simulink library "turbine_generator_v0"  (R2025b)
settings: Solver=VariableStepAuto  StartTime=0.0  StopTime=10.0  RelTol=1e-3
undefined symbols (not defined in the file): gen_eta, kT, kV, R_load, Rm, turbine_D
libraries: simulink x2
settings Model: Creator=Carson  LastModifiedBy=Carson
settings RTWCC: GPUComputeCapability=3.5

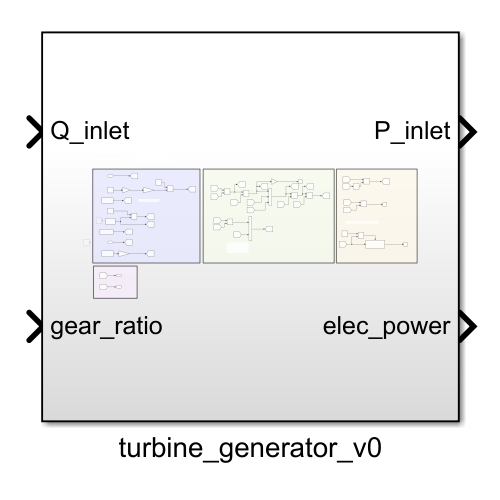
[thumbnail: Simulink's stored preview of the top-level diagram]
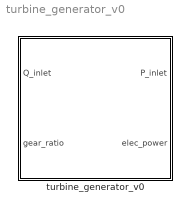
== system turbine_generator_v0 ==
  turbine_generator_v0 : Subsystem

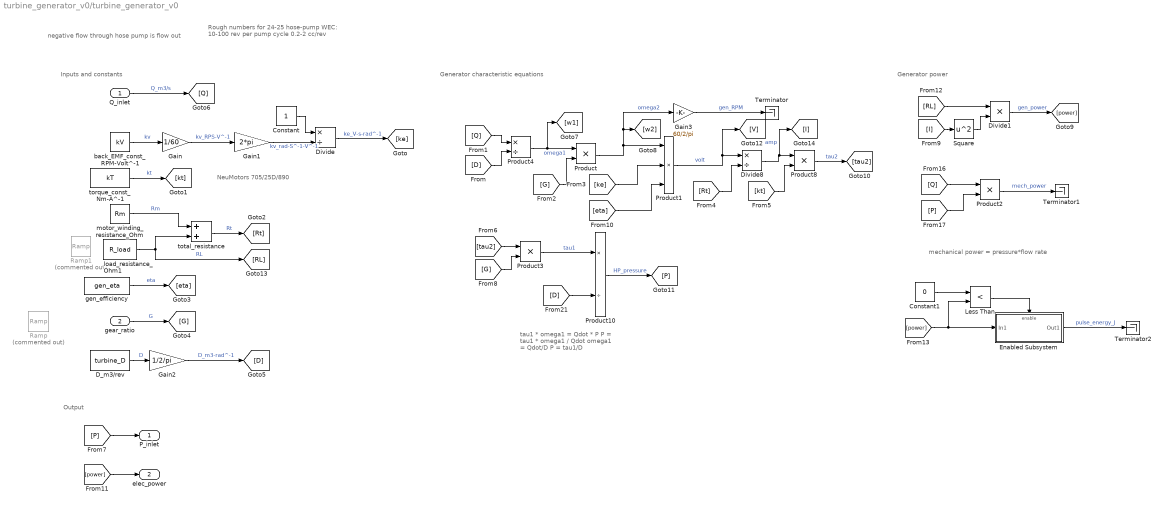
== system turbine_generator_v0/turbine_generator_v0 ==
  note: tau1 * omega1 = Qdot * P
      | P = tau1 * omega1 / Qdot
      | 	omega1 = Qdot/D
      | P = tau1/D
  note: NeuMotors 705/25D/890
  note: mechanical power = pressure*flow rate
  note: Rough numbers for 24-25 hose-pump WEC:
      | 	10-100 rev per pump cycle
      | 	0.2-2 cc/rev
  note: Generator power
  note: Output
  note: Generator characteristic equations
  note: Inputs and constants
  note: negative flow through hose pump is flow out
  Q_inlet : Inport
  gear_ratio : Inport  Port=2
  Constant : Constant
  Constant1 : Constant  Value=0
  D_m3/rev : Constant  Value=turbine_D
  Divide : Product  Inputs=*/
  Divide1 : Product  Inputs=**
  Divide8 : Product  Inputs=*/
  Enabled Subsystem : Subsystem  TreatAsAtomicUnit=on
  Gain : Gain  Gain=1/60
  Gain1 : Gain  Gain=2*pi
  Gain2 : Gain  Gain=1/2/pi
  Gain3 : Gain  Gain=60/2/pi
  Less Than : RelationalOperator  Operator=<  OutDataTypeStr=boolean  RndMeth=Simplest  InputSameDT=off
  Product{,2..3,8} (4 alike) : Product
  Product1 : Product  Inputs=3
  Product10 : Product  Inputs=*/
  Product4 : Product  Inputs=*/
  Ramp : simulink/Sources/Ramp  Commented=on  slope=0.1  start=60  InitialOutput=1
  Ramp1 : simulink/Sources/Ramp  Commented=on  slope=3/600  start=30  InitialOutput=0
  Square : Math  Operator=square
  Terminator : Terminator
  Terminator1 : Terminator
  Terminator2 : Terminator
  back_EMF_const_RPM-Volt^-1 : Constant  Value=kV
  gen_efficiency : Constant  Value=gen_eta
  load_resistance_Ohm1 : Constant  Value=R_load
  motor_winding_resistance_Ohm : Constant  Value=Rm
  torque_const_Nm-A^-1 : Constant  Value=kT
  total_resistance : Sum
  P_inlet : Outport
  elec_power : Outport  Port=2
  wires:
  torque_const_Nm-A^-1/1 -> [kt]  "kt"
  gen_efficiency/1 -> [eta]  "eta"
  motor_winding_resistance_Ohm/1 -> total_resistance/1  "Rm"
  load_resistance_Ohm1/1 -> total_resistance/2, [RL]  "RL"
  total_resistance/1 -> [Rt]  "Rt"
  Gain/1 -> Gain1/1  "kv_RPS-V^-1"
  Gain1/1 -> Divide/2  "kv_rad-S^-1-V^-1"
  Constant/1 -> Divide/1
  Divide/1 -> [ke]  "ke_V-s-rad^-1"
  D_m3/rev/1 -> Gain2/1  "D"
  Gain2/1 -> [D]  "D_m3-rad^-1"
  [P] -> P_inlet/1
  [RL] -> Divide1/1
  Divide1/1 -> [power]  "gen_power"
  [Q] -> Product2/1
  [P] -> Product2/2
  Product2/1 -> Terminator1/1  "mech_power"
  back_EMF_const_RPM-Volt^-1/1 -> Gain/1  "kv"
  gear_ratio/1 -> [G]  "G"
  [Q] -> Product4/1
  [D] -> Product4/2
  Product4/1 -> [w1], Product/1  "omega1"
  [G] -> Product/2
  Product/1 -> Gain3/1, [w2], Product1/1  "omega2"
  [ke] -> Product1/2
  Product1/1 -> [V], Divide8/1  "volt"
  [Rt] -> Divide8/2
  Divide8/1 -> [I], Product8/1  "amp"
  [kt] -> Product8/2
  Product8/1 -> [tau2]  "tau2"
  [tau2] -> Product3/1
  Product3/1 -> Product10/1  "tau1"
  [eta] -> Product1/3
  [D] -> Product10/2
  Product10/1 -> [P]  "HP_pressure"
  Q_inlet/1 -> [Q]  "Q_m3/s"
  [G] -> Product3/2
  Gain3/1 -> Terminator/1  "gen_RPM"
  [I] -> Square/1
  [power] -> elec_power/1
  Square/1 -> Divide1/2
  [power] -> Less Than/2, Enabled Subsystem/1(In1)
  Constant1/1 -> Less Than/1
  Less Than/1 -> Enabled Subsystem/Enable
  Enabled Subsystem/1(Out1) -> Terminator2/1  "pulse_energy_J"

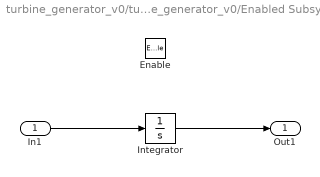
== system turbine_generator_v0/turbine_generator_v0/Enabled Subsystem ==
  In1 : Inport
  Enable : EnablePort  StatesWhenEnabling=reset
  Integrator : Integrator
  Out1 : Outport
  wires:
  In1/1 -> Integrator/1
  Integrator/1 -> Out1/1
